simulink model "FINN_MCI_Signal_Processing"  (R2020b)
settings: Solver=FixedStepDiscrete  StartTime=0.0  StopTime=SimTime  FixedStep=Ts_SIM  RelTol=1e-3
libraries: pdb_libbrowser x12
settings Model: Creator=BEDNASA  LastModifiedBy=HENRIE2

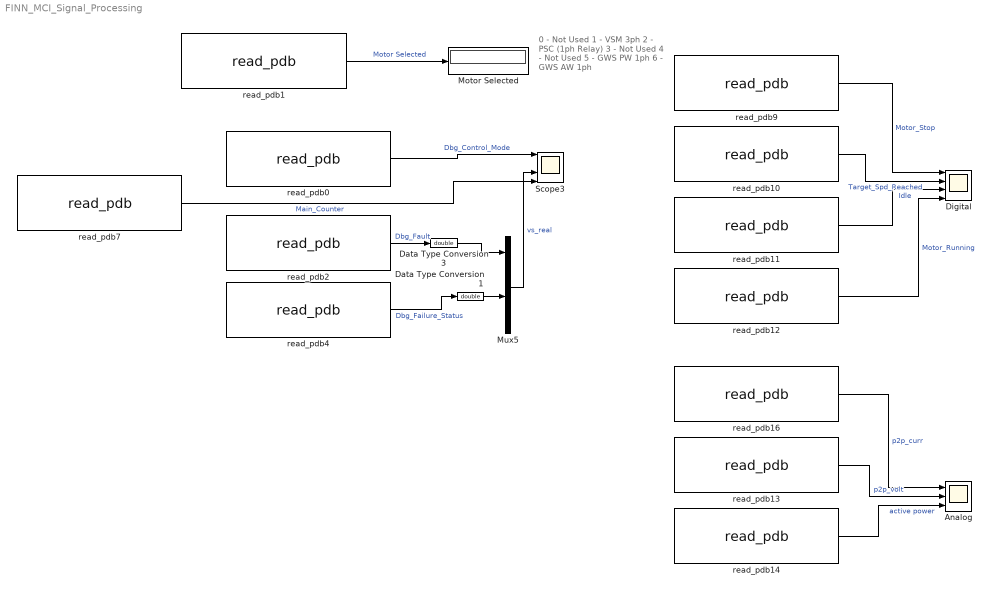
== system FINN_MCI_Signal_Processing ==
  note: 0 - Not Used
      | 1 - VSM 3ph
      | 2 - PSC (1ph Relay)
      | 3 - Not Used
      | 4 - Not Used
      | 5 - GWS PW 1ph
      | 6 - GWS AW 1ph
  Analog : Scope  NumInputPorts=3
  Data Type Conversion1 : DataTypeConversion  OutDataTypeStr=double
  Data Type Conversion3 : DataTypeConversion  OutDataTypeStr=double
  Digital : Scope  NumInputPorts=4
  Motor Selected : Display
  Mux5 : Mux
  Scope3 : Scope  NumInputPorts=4
  read_pdb0 : pdb_libbrowser/read_pdb  vstring=Dbg_Control_Mode
      settings: SourceProductName=Sim Arch
  read_pdb1 : pdb_libbrowser/read_pdb  vstring=Dbg_MciSlfac_Wash_Motor_Type
      settings: SourceProductName=Sim Arch
  read_pdb10 : pdb_libbrowser/read_pdb  vstring=My_GetDigital_1
      settings: SourceProductName=Sim Arch
  read_pdb11 : pdb_libbrowser/read_pdb  vstring=My_GetDigital_2
      settings: SourceProductName=Sim Arch
  read_pdb12 : pdb_libbrowser/read_pdb  vstring=My_GetDigital_3
      settings: SourceProductName=Sim Arch
  read_pdb13 : pdb_libbrowser/read_pdb  vstring=My_GetAnalog_1
      settings: SourceProductName=Sim Arch
  read_pdb14 : pdb_libbrowser/read_pdb  vstring=My_GetAnalog_2
      settings: SourceProductName=Sim Arch
  read_pdb16 : pdb_libbrowser/read_pdb  vstring=My_GetAnalog_0
      settings: SourceProductName=Sim Arch
  read_pdb2 : pdb_libbrowser/read_pdb  vstring=Dbg_MciSlfac_Last_Failure
      settings: SourceProductName=Sim Arch
  read_pdb4 : pdb_libbrowser/read_pdb  vstring=Dbg_Failure_State
      settings: SourceProductName=Sim Arch
  read_pdb7 : pdb_libbrowser/read_pdb  vstring=Dbg_Mcl_Main_Counter
      settings: SourceProductName=Sim Arch
  read_pdb9 : pdb_libbrowser/read_pdb  vstring=My_GetDigital_0
      settings: SourceProductName=Sim Arch
  wires:
  read_pdb1/1 -> Motor Selected/1  "Motor Selected"
  read_pdb0/1 -> Scope3/1  "Dbg_Control_Mode"
  Mux5/1 -> Scope3/3  "vs_real"
  Data Type Conversion1/1 -> Mux5/3
  read_pdb4/1 -> Data Type Conversion1/1  "Dbg_Failure_Status"
  read_pdb2/1 -> Data Type Conversion3/1  "Dbg_Fault"
  Data Type Conversion3/1 -> Mux5/1
  read_pdb7/1 -> Scope3/4  "Main_Counter"
  read_pdb9/1 -> Digital/1  "Motor_Stop"
  read_pdb10/1 -> Digital/2  "Target_Spd_Reached"
  read_pdb11/1 -> Digital/3  "Idle"
  read_pdb12/1 -> Digital/4  "Motor_Running"
  read_pdb16/1 -> Analog/1  "p2p_curr"
  read_pdb13/1 -> Analog/2  "p2p_volt"
  read_pdb14/1 -> Analog/3  "active power"
